simulink model "FindExactPosition"  (R2020b)
settings: Solver=VariableStepAuto  StartTime=0.0  StopTime=10.0  RelTol=1e-3
settings Model: Creator=macra  LastModifiedBy=macra

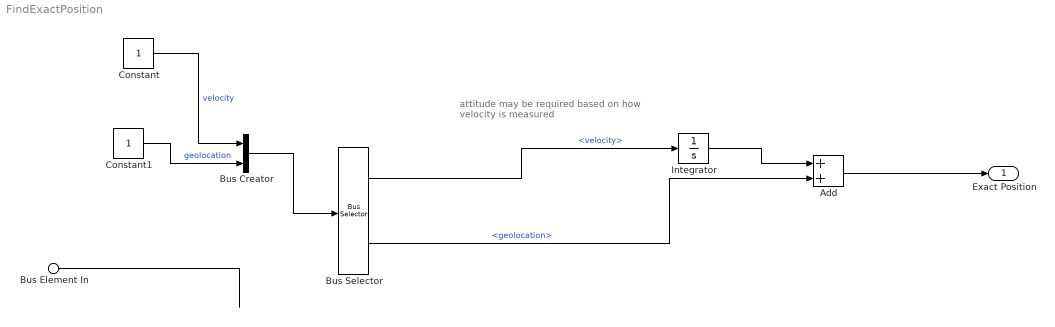
== system FindExactPosition ==
  note: attitude may be required based on how
      | velocity is measured
  Bus Element In : Inport  PortName=FlightData
  Add : Sum
  Bus Creator : BusCreator  Inputs=2
  Bus Selector : BusSelector  OutputSignals=velocity,geolocation
  Constant : Constant
  Constant1 : Constant
  Integrator : Integrator
  Exact Position : Outport
  wires:
  Bus Selector/2 -> Add/2  "<geolocation>"
  Bus Selector/1 -> Integrator/1  "<velocity>"
  Integrator/1 -> Add/1
  Add/1 -> Exact Position/1
  Bus Creator/1 -> Bus Selector/1
  Constant/1 -> Bus Creator/1  "velocity"
  Constant1/1 -> Bus Creator/2  "geolocation"
  Bus Element In/1 -> ?
